simulink model "rst_auto_reg_complete_2018b"  (R2018b)
settings: Solver=VariableStepAuto  StartTime=0.0  StopTime=100  RelTol=1e-3
values from neighbouring files (symbols this model uses):
  A = dend    [RST_2ordem_final.m]    (also in RST_4ordem_final.m)
  B = numd    [RST_2ordem_final.m]    (also in RST_4ordem_final.m)
  ep = 0.7    [RST_2ordem_final.m]    (also in RST_4ordem_final.m)
  initial_theta = [-0.31 -0.55 0.0021 0.12]    [RST_2ordem_final.m]    (also in RST_4ordem_final.m = [-1.0 0.38 0.07 0.23 0.03 0.12 0.06 0.005])
  Ta = 0.1    [RST_2ordem_final.m]    (also in RST_4ordem_final.m = 1)
  Tas = Ta    (= 0.1)    [RST_2ordem_final.m]    (also in RST_4ordem_final.m = 1)
  theta_switch_time = 10*Ta    (= 1)    [RST_2ordem_final.m]    (also in RST_4ordem_final.m = 10)
  Ts = 1    [RST_2ordem_final.m]    (also in RST_4ordem_final.m = 5)
  w0 = 1    [RST_2ordem_final.m]    (also in RST_4ordem_final.m = 0.1)
libraries: dspinverses x6, simulink x1
settings Model: Creator=tarci  LastModifiedBy=root
settings DebuggingCC: LibraryContextMissingDiagnostic=none
settings SFSimCC: SimUseLocalCustomCode=off
settings RTWCC: RTWUseLocalCustomCode=off

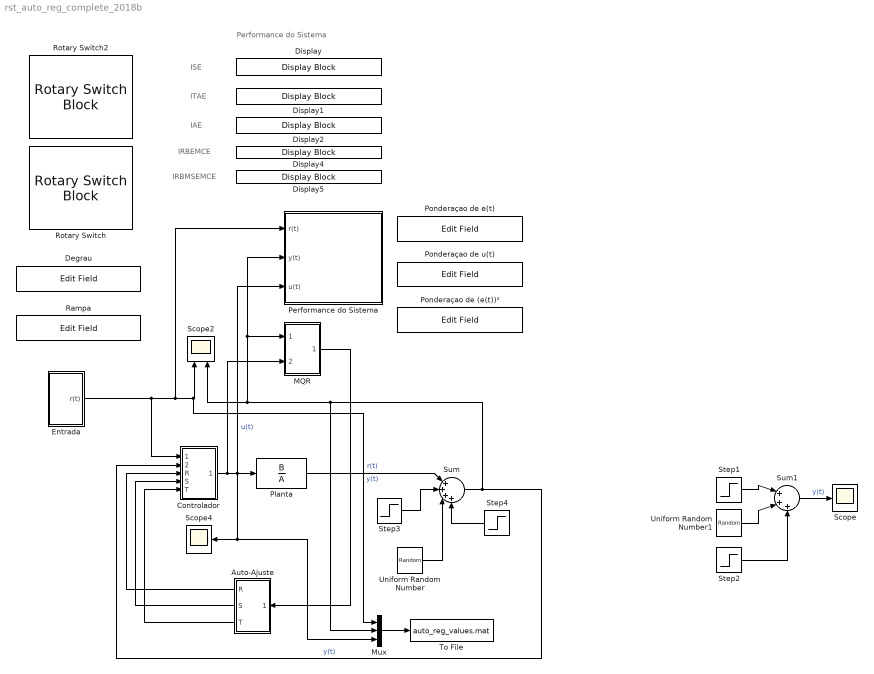
== system rst_auto_reg_complete_2018b ==
  note: ISE
  note: Performance do Sistema
  note: ITAE
  note: IAE
  note: IRBEMCE
  note: IRBMSEMCE
  Auto-Ajuste : Subsystem
  Controlador : Subsystem
  Degrau : EditField  WebBlockId=1122  LabelPosition=Hide  ShowInitialText=on  Alignment=Center
  Display : DisplayBlock  WebBlockId=1210  LabelPosition=Hide
  Display1 : DisplayBlock  WebBlockId=1211  LabelPosition=Hide
  Display2 : DisplayBlock  WebBlockId=1212  LabelPosition=Hide
  Display4 : DisplayBlock  WebBlockId=1214  LabelPosition=Hide
  Display5 : DisplayBlock  WebBlockId=1215  LabelPosition=Hide
  Entrada : Subsystem
  MQR : Subsystem
  Mux : Mux  Inputs=3
  Performance do Sistema : Subsystem
  Planta : DiscreteFilter  Numerator=B  Denominator=A  SampleTime=Ta  a0EqualsOne=on
  Ponderaçao de (e(t))² : EditField  WebBlockId=1158  LabelPosition=Hide  ShowInitialText=on  Alignment=Center
  Ponderaçao de e(t) : EditField  WebBlockId=1155  LabelPosition=Hide  ShowInitialText=on  Alignment=Center
  Ponderaçao de u(t) : EditField  WebBlockId=1156  LabelPosition=Hide  ShowInitialText=on  Alignment=Center
  Rampa : EditField  WebBlockId=1123  LabelPosition=Hide  ShowInitialText=on  Alignment=Center
  Rotary Switch : RotarySwitchBlock  WebBlockId=1169
      settings: Values={{'Degrau', 'Rampa', 'Senoide'}, [1 2 3]}
  Rotary Switch2 : RotarySwitchBlock  WebBlockId=1120
      settings: Values={{'Degrau', 'Rampa', 'Senoide'}, [1 2 3]}
  Scope : Scope
  Scope2 : Scope  NumInputPorts=2
  Scope4 : Scope
  Step1 : Step  Time=60  SampleTime=0
  Step2 : Step  Time=61  After=-1  SampleTime=0
  Step3 : Step  Time=60  SampleTime=0
  Step4 : Step  Time=61  After=-1  SampleTime=0
  Sum : Sum  Inputs=|++++
  Sum1 : Sum  Inputs=|+++
  To File : ToFile  Filename=auto_reg_values.mat
  Uniform Random Number : UniformRandomNumber  Minimum=-0.10  Maximum=0.10  Seed=10  SampleTime=0
  Uniform Random Number1 : UniformRandomNumber  Minimum=-0.10  Maximum=0.10  Seed=10  SampleTime=0
  wires:
  Auto-Ajuste/3(T) -> Controlador/5(T)
  Auto-Ajuste/1(R) -> Controlador/3(R)
  MQR/1("Theta(t) ") -> Auto-Ajuste/1(Theta)
  Entrada/1(r(t)) -> Mux/1, Scope2/1, Performance do Sistema/1(r(t)), Controlador/1(r(t))  "r(t)"
  Controlador/1(u(t)) -> Mux/3, Scope4/1, Performance do Sistema/3(u(t)), Planta/1, MQR/2("u(t) ")  "u(t)"
  Auto-Ajuste/2(S) -> Controlador/4(S)
  Mux/1 -> To File/1
  Step3/1 -> Sum/2
  Uniform Random Number/1 -> Sum/3
  Step4/1 -> Sum/4
  Planta/1 -> Sum/1  "y(t)"
  Sum/1 -> Mux/2, Scope2/2, Performance do Sistema/2(y(t)), MQR/1(y(t)), Controlador/2(y(t))  "y(t)"
  Uniform Random Number1/1 -> Sum1/2
  Step2/1 -> Sum1/3
  Step1/1 -> Sum1/1
  Sum1/1 -> Scope/1  "y(t)"

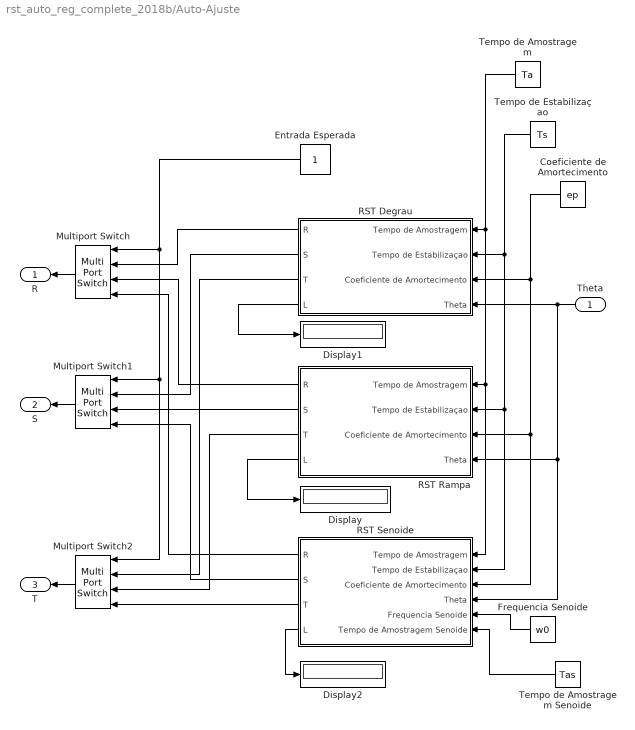
== system rst_auto_reg_complete_2018b/Auto-Ajuste ==
  Theta : Inport
  Coeficiente de Amortecimento : Constant  Value=ep
  Display : Display
  Display1 : Display
  Display2 : Display
  Entrada Esperada : Constant
  Frequencia Senoide : Constant  Value=w0
  Multiport Switch : MultiPortSwitch
  Multiport Switch1 : MultiPortSwitch
  Multiport Switch2 : MultiPortSwitch
  RST Degrau : Subsystem
  RST Rampa : Subsystem
  RST Senoide : Subsystem
  Tempo de Amostragem : Constant  Value=Ta
  Tempo de Amostragem Senoide : Constant  Value=Tas
  Tempo de Estabilizaçao : Constant  Value=Ts
  R : Outport
  S : Outport  Port=2
  T : Outport  Port=3
  wires:
  Entrada Esperada/1 -> Multiport Switch1/1, Multiport Switch2/1, Multiport Switch/1
  RST Degrau/1(R) -> Multiport Switch/2
  Coeficiente de Amortecimento/1 -> RST Senoide/3(Coeficiente de Amortecimento), RST Rampa/3(Coeficiente de Amortecimento), RST Degrau/3(Coeficiente de Amortecimento)
  RST Degrau/3(T) -> Multiport Switch2/2
  Theta/1 -> RST Senoide/4(Theta), RST Rampa/4(Theta), RST Degrau/4(Theta)
  RST Rampa/3(T) -> Multiport Switch2/3
  Tempo de Amostragem/1 -> RST Senoide/1(Tempo de Amostragem), RST Rampa/1(Tempo de Amostragem), RST Degrau/1(Tempo de Amostragem)
  Tempo de Amostragem Senoide/1 -> RST Senoide/6(Tempo de Amostragem Senoide)
  Frequencia Senoide/1 -> RST Senoide/5(Frequencia Senoide)
  RST Rampa/1(R) -> Multiport Switch/3
  RST Senoide/2(S) -> Multiport Switch1/4
  RST Degrau/2(S) -> Multiport Switch1/2
  Tempo de Estabilizaçao/1 -> RST Senoide/2(Tempo de Estabilizaçao), RST Rampa/2(Tempo de Estabilizaçao), RST Degrau/2(Tempo de Estabilizaçao)
  RST Senoide/1(R) -> Multiport Switch/4
  Multiport Switch/1 -> R/1
  Multiport Switch1/1 -> S/1
  Multiport Switch2/1 -> T/1
  RST Rampa/4(L) -> Display/1
  RST Senoide/3(T) -> Multiport Switch2/4
  RST Rampa/2(S) -> Multiport Switch1/3
  RST Degrau/4(L) -> Display1/1
  RST Senoide/4(L) -> Display2/1

== system rst_auto_reg_complete_2018b/Controlador ==
  r(t) : Inport
  y(t) : Inport  Port=2
  R : Inport  Port=3
  S : Inport  Port=4
  T : Inport  Port=5
  1/S3 : DiscreteFilter  Numerator=1  DenominatorSource=Input port  Denominator=1  SampleTime=Ta  a0EqualsOne=on
      settings: InputPortMap=u0,p3
  R3 : DiscreteFilter  NumeratorSource=Input port  Numerator=[-620.2 131.3]  Denominator=1  SampleTime=Ta
      settings: InputPortMap=u0,p1
  Sum11 : Sum  Inputs=|+-
  T3 : DiscreteFilter  NumeratorSource=Input port  Numerator=13.39  Denominator=1  SampleTime=Ta
      settings: InputPortMap=u0,p1
  u(t) : Outport
  wires:
  T3/1 -> Sum11/1
  T/1 -> T3/2
  Sum11/1 -> 1/S3/1
  R3/1 -> Sum11/2
  R/1 -> R3/2
  S/1 -> 1/S3/2
  r(t)/1 -> T3/1
  y(t)/1 -> R3/1
  1/S3/1 -> u(t)/1  "u(t)"

== system rst_auto_reg_complete_2018b/Entrada ==
  Multiport Switch : MultiPortSwitch
  Ramp : simulink/Sources/Ramp  slope=1  start=0  InitialOutput=0
  Sine Wave : Sin  Frequency=w0  SampleTime=Tas
  Step1 : Step  Time=0  SampleTime=0
  Step2 : Step  Time=10  After=2  SampleTime=0
  Step3 : Step  Time=20  After=-3  SampleTime=0
  Step4 : Step  Time=30  After=4  SampleTime=0
  Step5 : Step  Time=50  After=-2  SampleTime=0
  Sum : Sum  Inputs=|+++++
  Tipo de Entrada : Constant
  r(t) : Outport
  wires:
  Sine Wave/1 -> Multiport Switch/4
  Ramp/1 -> Multiport Switch/3
  Tipo de Entrada/1 -> Multiport Switch/1
  Multiport Switch/1 -> r(t)/1
  Step1/1 -> Sum/1
  Step2/1 -> Sum/2
  Step3/1 -> Sum/3
  Step4/1 -> Sum/4
  Sum/1 -> Multiport Switch/2
  Step5/1 -> Sum/5

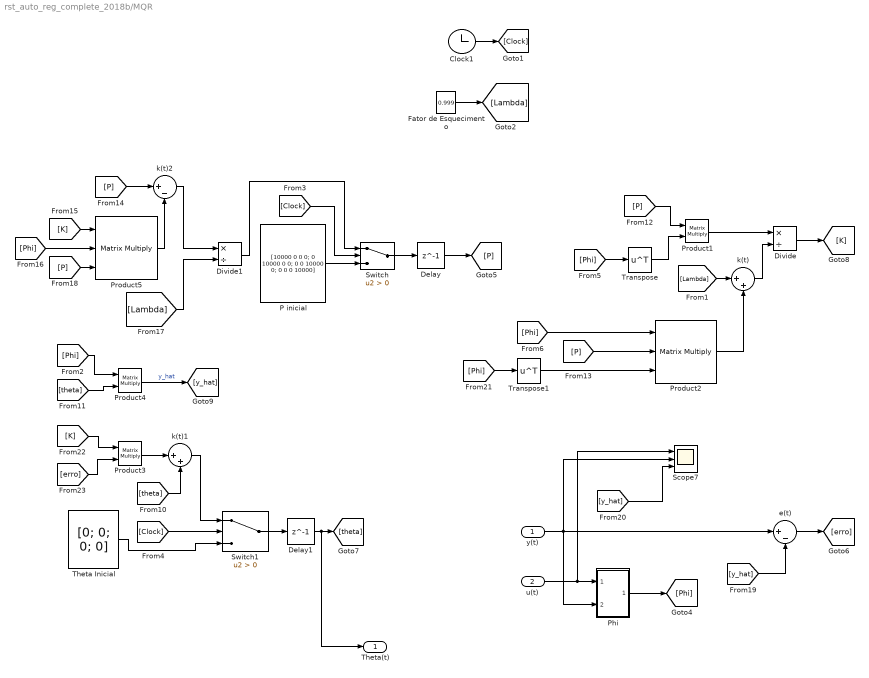
== system rst_auto_reg_complete_2018b/MQR ==
  y(t) : Inport
  "u(t) " : Inport  Port=2
  Clock1 : Clock
  Delay : Delay  DelayLength=1  InitialCondition=0
  Delay1 : Delay  DelayLength=1  InitialCondition=0
  Divide : Product  Inputs=*/
  Divide1 : Product  Inputs=*/
  "Fator de Esquecimento " : Constant  Value=0.999
  P inicial : Constant  Value=[10000 0 0 0; 0 10000 0 0; 0 0 10000 0; 0 0 0 10000]
  Phi : Subsystem
  Product1 : Product  Multiplication=Matrix(*)
  Product2 : Product  Inputs=3  Multiplication=Matrix(*)
  Product3 : Product  Multiplication=Matrix(*)
  Product4 : Product  Multiplication=Matrix(*)
  Product5 : Product  Inputs=3  Multiplication=Matrix(*)
  Scope7 : Scope  NumInputPorts=3
  Switch : Switch  Criteria=u2 > Threshold
  Switch1 : Switch  Criteria=u2 > Threshold
  "Theta Inicial " : Constant  Value=[0; 0; 0; 0]
  Transpose : Math  Operator=transpose  SaturateOnIntegerOverflow=on
  Transpose1 : Math  Operator=transpose  SaturateOnIntegerOverflow=on
  e(t) : Sum  Inputs=|+-
  k(t) : Sum  Inputs=|++
  k(t)1 : Sum  Inputs=|++
  k(t)2 : Sum  Inputs=|+-
  "Theta(t) " : Outport
  wires:
  k(t)/1 -> Divide/2
  [Phi] -> Product4/1
  Phi/1(Phi) -> [Phi]
  k(t)1/1 -> Switch1/1
  [y_hat] -> Scope7/3
  Switch1/1 -> Delay1/1
  [K] -> Product3/1
  Product2/1 -> k(t)/2
  [Clock] -> Switch1/2
  y(t)/1 -> e(t)/1, Scope7/2, Phi/2(y(t))
  k(t)2/1 -> Divide1/1
  Delay1/1 -> "Theta(t) "/1, [theta]
  Product5/1 -> k(t)2/2
  "u(t) "/1 -> Scope7/1, Phi/1(u(t))
  Switch/1 -> Delay/1
  [Lambda] -> Divide1/2
  Product1/1 -> Divide/1
  e(t)/1 -> [erro]
  Product3/1 -> k(t)1/1
  Delay/1 -> [P]
  [Phi] -> Transpose1/1
  [P] -> Product5/3
  "Fator de Esquecimento "/1 -> [Lambda]
  "Theta Inicial "/1 -> Switch1/3
  Transpose1/1 -> Product2/3
  Divide1/1 -> Switch/1
  [Phi] -> Transpose/1
  [Clock] -> Switch/2
  [theta] -> Product4/2
  [P] -> k(t)2/1
  [theta] -> k(t)1/2
  [P] -> Product2/2
  [Lambda] -> k(t)/1
  Transpose/1 -> Product1/2
  Clock1/1 -> [Clock]
  [erro] -> Product3/2
  [y_hat] -> e(t)/2
  [K] -> Product5/1
  P inicial/1 -> Switch/3
  [P] -> Product1/1
  [Phi] -> Product2/1
  Divide/1 -> [K]
  [Phi] -> Product5/2
  Product4/1 -> [y_hat]  "y_hat"

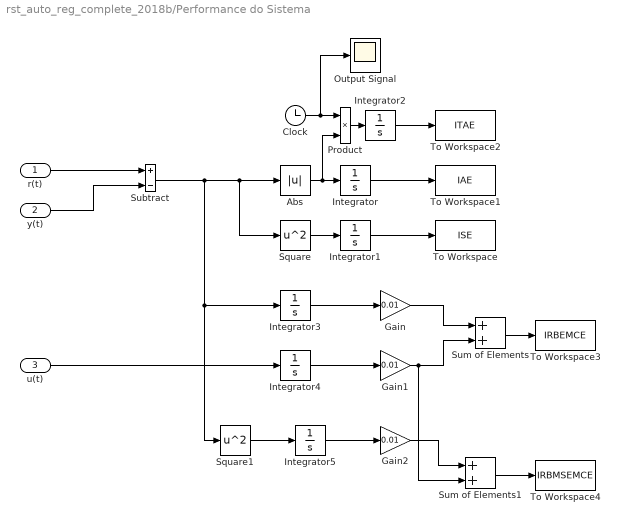
== system rst_auto_reg_complete_2018b/Performance do Sistema ==
  r(t) : Inport
  y(t) : Inport  Port=2
  u(t) : Inport  Port=3
  Abs : Abs
  Clock : Clock
  Gain : Gain  Gain=0.01
  Gain1 : Gain  Gain=0.01
  Gain2 : Gain  Gain=0.01
  Integrator{,1..5} (6 alike) : Integrator
  Output Signal : Scope
  Product : Product
  Square : Math  Operator=square  SaturateOnIntegerOverflow=on
  Square1 : Math  Operator=square  SaturateOnIntegerOverflow=on
  Subtract : Sum  Inputs=+-
  Sum of Elements : Sum
  Sum of Elements1 : Sum
  To Workspace : ToWorkspace  VariableName=ISE  SaveFormat=Timeseries  SampleTime=-1
  To Workspace1 : ToWorkspace  VariableName=IAE  SaveFormat=Timeseries  SampleTime=-1
  To Workspace2 : ToWorkspace  VariableName=ITAE  SaveFormat=Timeseries  SampleTime=-1
  To Workspace3 : ToWorkspace  VariableName=IRBEMCE  SaveFormat=Timeseries  SampleTime=-1
  To Workspace4 : ToWorkspace  VariableName=IRBMSEMCE  SaveFormat=Timeseries  SampleTime=-1
  wires:
  y(t)/1 -> Subtract/2
  Abs/1 -> Product/2, Integrator/1
  Integrator/1 -> To Workspace1/1
  Integrator1/1 -> To Workspace/1
  Square/1 -> Integrator1/1
  Clock/1 -> Output Signal/1, Product/1
  Product/1 -> Integrator2/1
  Integrator2/1 -> To Workspace2/1
  r(t)/1 -> Subtract/1
  Subtract/1 -> Square1/1, Integrator3/1, Square/1, Abs/1
  Integrator3/1 -> Gain/1
  Integrator4/1 -> Gain1/1
  Gain/1 -> Sum of Elements/1
  Gain1/1 -> Sum of Elements1/2, Sum of Elements/2
  Square1/1 -> Integrator5/1
  Integrator5/1 -> Gain2/1
  Gain2/1 -> Sum of Elements1/1
  Sum of Elements/1 -> To Workspace3/1
  Sum of Elements1/1 -> To Workspace4/1
  u(t)/1 -> Integrator4/1

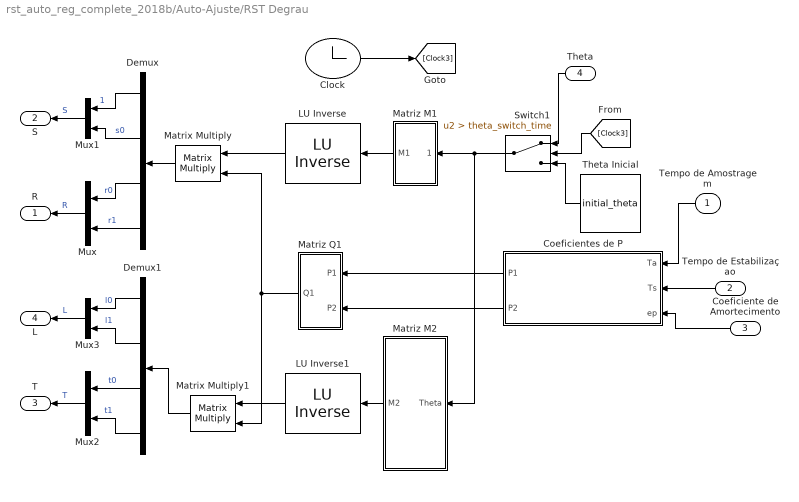
== system rst_auto_reg_complete_2018b/Auto-Ajuste/RST Degrau ==
  Tempo de Amostragem : Inport
  Tempo de Estabilizaçao : Inport  Port=2
  Coeficiente de Amortecimento : Inport  Port=3
  Theta : Inport  Port=4
  " LU Inverse" : dspinverses/ LU Inverse
      settings: SourceProductName=DSP System Toolbox
  " LU Inverse1" : dspinverses/ LU Inverse
      settings: SourceProductName=DSP System Toolbox
  Clock : Clock
  Coeficientes de P : Subsystem
  Demux : Demux
  Demux1 : Demux
  Matrix Multiply : Product  Multiplication=Matrix(*)
  Matrix Multiply1 : Product  Multiplication=Matrix(*)
  Matriz M1 : Subsystem
  Matriz M2 : Subsystem
  Matriz Q1 : Subsystem
  Mux{,1..3} (4 alike) : Mux  Inputs=2
  Switch1 : Switch  Criteria=u2 > Threshold  Threshold=theta_switch_time
  Theta Inicial : Constant  Value=initial_theta
  R : Outport
  S : Outport  Port=2
  T : Outport  Port=3
  L : Outport  Port=4
  wires:
  Matrix Multiply/1 -> Demux/1
  " LU Inverse"/1 -> Matrix Multiply/1
  Mux1/1 -> S/1  "S"
  Coeficientes de P/2(P2) -> Matriz Q1/2(P2)
  Tempo de Estabilizaçao/1 -> Coeficientes de P/2(Ts)
  Coeficiente de Amortecimento/1 -> Coeficientes de P/3(ep)
  Tempo de Amostragem/1 -> Coeficientes de P/1(Ta)
  Coeficientes de P/1(P1) -> Matriz Q1/1(P1)
  Mux/1 -> R/1  "R"
  Clock/1 -> [Clock3]
  Switch1/1 -> Matriz M2/1(Theta), Matriz M1/1(In1)
  Theta/1 -> Switch1/1
  [Clock3] -> Switch1/2
  Theta Inicial/1 -> Switch1/3
  Matriz M1/1(M1) -> " LU Inverse"/1
  Demux/1 -> Mux1/1  "1"
  Demux/2 -> Mux1/2  "s0"
  Demux/3 -> Mux/1  "r0"
  Demux/4 -> Mux/2  "r1"
  " LU Inverse1"/1 -> Matrix Multiply1/1
  Matriz Q1/1(Q1) -> Matrix Multiply/2, Matrix Multiply1/2
  Matriz M2/1(M2) -> " LU Inverse1"/1
  Demux1/3 -> Mux2/1  "t0"
  Mux2/1 -> T/1  "T"
  Demux1/2 -> Mux3/2  "l1"
  Mux3/1 -> L/1  "L"
  Demux1/1 -> Mux3/1  "l0"
  Matrix Multiply1/1 -> Demux1/1
  Demux1/4 -> Mux2/2  "t1"

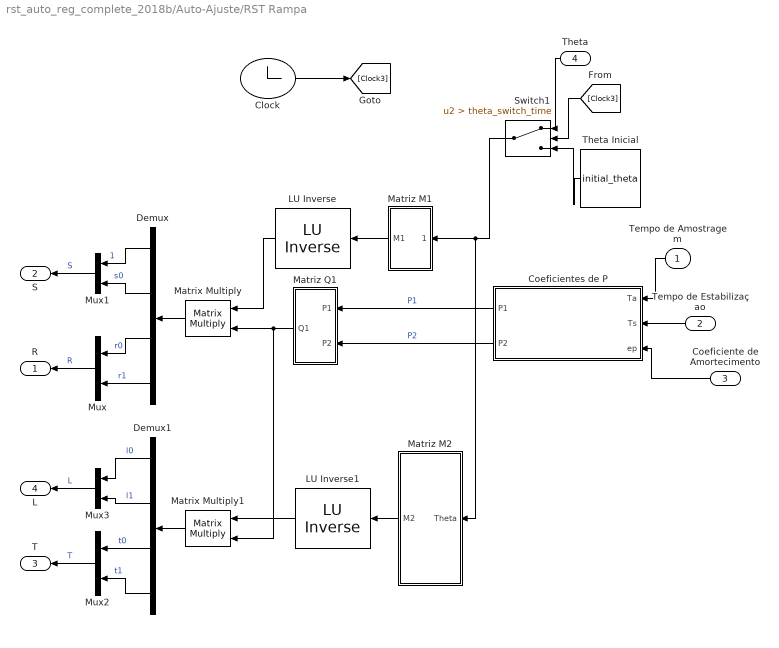
== system rst_auto_reg_complete_2018b/Auto-Ajuste/RST Rampa ==
  Tempo de Amostragem : Inport
  Tempo de Estabilizaçao : Inport  Port=2
  Coeficiente de Amortecimento : Inport  Port=3
  Theta : Inport  Port=4
  " LU Inverse" : dspinverses/ LU Inverse
      settings: SourceProductName=DSP System Toolbox
  " LU Inverse1" : dspinverses/ LU Inverse
      settings: SourceProductName=DSP System Toolbox
  Clock : Clock
  Coeficientes de P : Subsystem
  Demux : Demux
  Demux1 : Demux
  Matrix Multiply : Product  Multiplication=Matrix(*)
  Matrix Multiply1 : Product  Multiplication=Matrix(*)
  Matriz M1 : Subsystem
  Matriz M2 : Subsystem
  Matriz Q1 : Subsystem
  Mux{,1..3} (4 alike) : Mux  Inputs=2
  Switch1 : Switch  Criteria=u2 > Threshold  Threshold=theta_switch_time
  Theta Inicial : Constant  Value=initial_theta
  R : Outport
  S : Outport  Port=2
  T : Outport  Port=3
  L : Outport  Port=4
  wires:
  Demux/4 -> Mux/2  "r1"
  Demux/3 -> Mux/1  "r0"
  Demux/2 -> Mux1/2  "s0"
  Demux/1 -> Mux1/1  "1"
  Matriz Q1/1(Q1) -> Matrix Multiply/2, Matrix Multiply1/2
  Matriz M1/1(M1) -> " LU Inverse"/1
  Theta Inicial/1 -> Switch1/3
  [Clock3] -> Switch1/2
  Theta/1 -> Switch1/1
  Switch1/1 -> Matriz M2/1(Theta), Matriz M1/1(In1)
  Clock/1 -> [Clock3]
  Mux/1 -> R/1  "R"
  Coeficientes de P/1(P1) -> Matriz Q1/1(P1)  "P1"
  Tempo de Amostragem/1 -> Coeficientes de P/1(Ta)
  Coeficiente de Amortecimento/1 -> Coeficientes de P/3(ep)
  Tempo de Estabilizaçao/1 -> Coeficientes de P/2(Ts)
  Coeficientes de P/2(P2) -> Matriz Q1/2(P2)  "P2"
  Mux1/1 -> S/1  "S"
  " LU Inverse"/1 -> Matrix Multiply/1
  Matrix Multiply/1 -> Demux/1
  Matriz M2/1(M2) -> " LU Inverse1"/1
  " LU Inverse1"/1 -> Matrix Multiply1/1
  Mux3/1 -> L/1  "L"
  Mux2/1 -> T/1  "T"
  Demux1/1 -> Mux3/1  "l0"
  Demux1/2 -> Mux3/2  "l1"
  Demux1/3 -> Mux2/1  "t0"
  Demux1/4 -> Mux2/2  "t1"
  Matrix Multiply1/1 -> Demux1/1

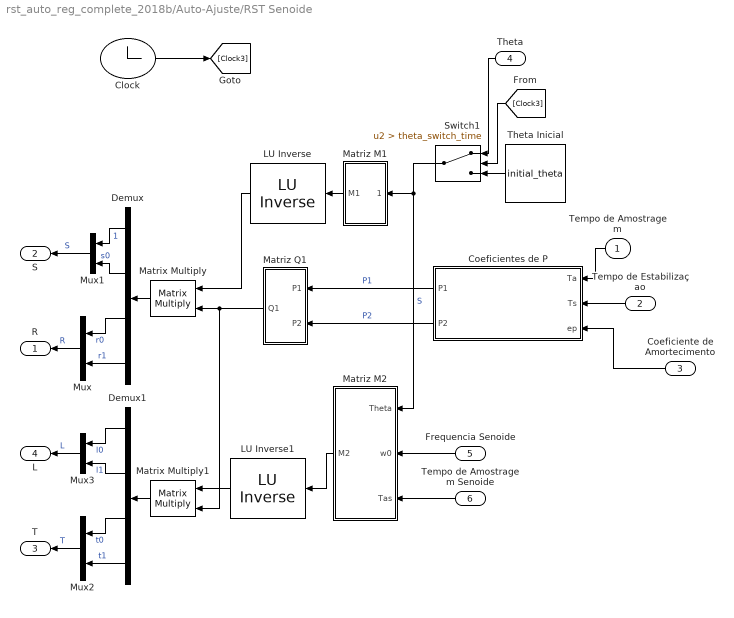
== system rst_auto_reg_complete_2018b/Auto-Ajuste/RST Senoide ==
  Tempo de Amostragem : Inport
  Tempo de Estabilizaçao : Inport  Port=2
  Coeficiente de Amortecimento : Inport  Port=3
  Theta : Inport  Port=4
  Frequencia Senoide : Inport  Port=5
  Tempo de Amostragem Senoide : Inport  Port=6
  " LU Inverse" : dspinverses/ LU Inverse
      settings: SourceProductName=DSP System Toolbox
  " LU Inverse1" : dspinverses/ LU Inverse
      settings: SourceProductName=DSP System Toolbox
  Clock : Clock
  Coeficientes de P : Subsystem
  Demux : Demux
  Demux1 : Demux
  Matrix Multiply : Product  Multiplication=Matrix(*)
  Matrix Multiply1 : Product  Multiplication=Matrix(*)
  Matriz M1 : Subsystem
  Matriz M2 : Subsystem
  Matriz Q1 : Subsystem
  Mux{,1..3} (4 alike) : Mux  Inputs=2
  Switch1 : Switch  Criteria=u2 > Threshold  Threshold=theta_switch_time
  Theta Inicial : Constant  Value=initial_theta
  R : Outport
  S : Outport  Port=2
  T : Outport  Port=3
  L : Outport  Port=4
  wires:
  Demux/4 -> Mux/2  "r1"
  Demux/3 -> Mux/1  "r0"
  Demux/2 -> Mux1/2  "s0"
  Demux/1 -> Mux1/1  "1"
  Matriz Q1/1(Q1) -> Matrix Multiply/2, Matrix Multiply1/2
  Matriz M1/1(M1) -> " LU Inverse"/1
  Theta Inicial/1 -> Switch1/3
  [Clock3] -> Switch1/2
  Theta/1 -> Switch1/1
  Switch1/1 -> Matriz M2/1(Theta), Matriz M1/1(In1)  "S"
  Clock/1 -> [Clock3]
  Mux/1 -> R/1  "R"
  Coeficientes de P/1(P1) -> Matriz Q1/1(P1)  "P1"
  Tempo de Amostragem/1 -> Coeficientes de P/1(Ta)
  Coeficiente de Amortecimento/1 -> Coeficientes de P/3(ep)
  Tempo de Estabilizaçao/1 -> Coeficientes de P/2(Ts)
  Coeficientes de P/2(P2) -> Matriz Q1/2(P2)  "P2"
  Mux1/1 -> S/1  "S"
  " LU Inverse"/1 -> Matrix Multiply/1
  Matrix Multiply/1 -> Demux/1
  Frequencia Senoide/1 -> Matriz M2/2(w0)
  Tempo de Amostragem Senoide/1 -> Matriz M2/3(Tas)
  Matriz M2/1(M2) -> " LU Inverse1"/1
  " LU Inverse1"/1 -> Matrix Multiply1/1
  Mux3/1 -> L/1  "L"
  Mux2/1 -> T/1  "T"
  Demux1/1 -> Mux3/1  "l0"
  Demux1/2 -> Mux3/2  "l1"
  Demux1/3 -> Mux2/1  "t0"
  Demux1/4 -> Mux2/2  "t1"
  Matrix Multiply1/1 -> Demux1/1

== system rst_auto_reg_complete_2018b/MQR/Phi ==
  u(t) : Inport
  y(t) : Inport  Port=2
  Constant : Constant  Value=-1
  Delay : Delay
  Delay1 : Delay  DelayLength=1
  Delay2 : Delay
  Delay3 : Delay  DelayLength=1
  Product : Product
  Transpose1 : Math  Operator=transpose  SaturateOnIntegerOverflow=on
  Vector Concatenate : Concatenate  NumInputs=4
  Phi : Outport
  wires:
  u(t)/1 -> Delay2/1, Delay3/1
  Vector Concatenate/1 -> Transpose1/1  "Phi"
  Delay/1 -> Vector Concatenate/2
  y(t)/1 -> Product/1
  Delay3/1 -> Vector Concatenate/3
  Delay2/1 -> Vector Concatenate/4
  Delay1/1 -> Vector Concatenate/1
  Transpose1/1 -> Phi/1
  Constant/1 -> Product/2
  Product/1 -> Delay/1, Delay1/1

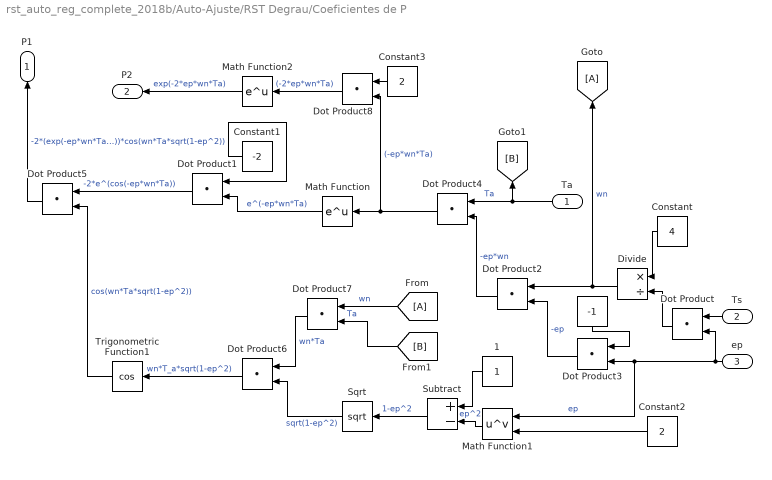
== system rst_auto_reg_complete_2018b/Auto-Ajuste/RST Degrau/Coeficientes de P ==
  Ta : Inport
  Ts : Inport  Port=2
  ep : Inport  Port=3
  " " : Constant  Value=-1
  1 : Constant
  Constant : Constant  Value=4
  Constant1 : Constant  Value=-2
  Constant2 : Constant  Value=2
  Constant3 : Constant  Value=2
  Divide : Product  Inputs=*/
  Dot Product{,1..8} (9 alike) : DotProduct  InputSameDT=on  OutDataTypeStr=Inherit: Inherit via internal rule
  Math Function : Math  SaturateOnIntegerOverflow=on
  Math Function1 : Math  Operator=pow  SaturateOnIntegerOverflow=on
  Math Function2 : Math  SaturateOnIntegerOverflow=on
  Sqrt : Sqrt  SaturateOnIntegerOverflow=on
  Subtract : Sum  Inputs=+-
  Trigonometric Function1 : Trigonometry  Operator=cos
  P1 : Outport
  P2 : Outport  Port=2
  wires:
  Math Function/1 -> Dot Product1/2  "e^(-ep*wn*Ta)"
  Divide/1 -> Dot Product2/1, [A]  "wn"
  [A] -> Dot Product7/1  "wn"
  " "/1 -> Dot Product3/1
  Dot Product5/1 -> P1/1  "-2*(exp(-ep*wn*Ta))*cos(wn*Ta*sqrt(1-ep^2))"
  Trigonometric Function1/1 -> Dot Product5/2  "cos(wn*Ta*sqrt(1-ep^2))"
  Ts/1 -> Dot Product/1
  Dot Product/1 -> Divide/2
  Dot Product3/1 -> Dot Product2/2  "-ep"
  ep/1 -> Math Function1/1, Dot Product3/2, Dot Product/2  "ep"
  Constant/1 -> Divide/1
  Dot Product7/1 -> Dot Product6/1  "wn*Ta"
  Ta/1 -> Dot Product4/1, [B]  "Ta"
  Math Function1/1 -> Subtract/2  "ep^2"
  Dot Product1/1 -> Dot Product5/1  "-2*e^(cos(-ep*wn*Ta))"
  Constant2/1 -> Math Function1/2
  1/1 -> Subtract/1
  Constant1/1 -> Dot Product1/1
  Dot Product2/1 -> Dot Product4/2  "-ep*wn"
  [B] -> Dot Product7/2  "Ta"
  Dot Product6/1 -> Trigonometric Function1/1  "wn*T_a*sqrt(1-ep^2)"
  Dot Product4/1 -> Dot Product8/2, Math Function/1  "(-ep*wn*Ta)"
  Sqrt/1 -> Dot Product6/2  "sqrt(1-ep^2)"
  Subtract/1 -> Sqrt/1  "1-ep^2"
  Constant3/1 -> Dot Product8/1
  Dot Product8/1 -> Math Function2/1  "(-2*ep*wn*Ta)"
  Math Function2/1 -> P2/1  "exp(-2*ep*wn*Ta)"

== system rst_auto_reg_complete_2018b/Auto-Ajuste/RST Degrau/Matriz M1 ==
  In1 : Inport
  " 1" : Constant  Value=0
  2 : Constant
  Demux : Demux
  Matrix Concatenate{6,9..11} (4 alike) : Concatenate  NumInputs=4  Mode=Multidimensional array  ConcatenateDimension=2
  Matrix Concatenate12 : Concatenate  Mode=Multidimensional array
  Matrix Concatenate13 : Concatenate  Mode=Multidimensional array
  Matrix Concatenate14 : Concatenate  Mode=Multidimensional array
  M1 : Outport
  wires:
  In1/1 -> Demux/1
  Demux/3 -> Matrix Concatenate9/3, Matrix Concatenate10/4  "b1"
  Matrix Concatenate14/1 -> M1/1
  Demux/1 -> Matrix Concatenate10/2, Matrix Concatenate9/1  "a1"
  Demux/4 -> Matrix Concatenate10/3, Matrix Concatenate11/4  "b2"
  Demux/2 -> Matrix Concatenate11/2, Matrix Concatenate10/1  "a2"
  2/1 -> Matrix Concatenate9/2, Matrix Concatenate6/1  "1"
  " 1"/1 -> Matrix Concatenate6/3, Matrix Concatenate11/3, Matrix Concatenate11/1, Matrix Concatenate9/4, Matrix Concatenate6/4, Matrix Concatenate6/2  "0"
  Matrix Concatenate6/1 -> Matrix Concatenate12/1
  Matrix Concatenate9/1 -> Matrix Concatenate12/2
  Matrix Concatenate10/1 -> Matrix Concatenate13/1
  Matrix Concatenate11/1 -> Matrix Concatenate13/2
  Matrix Concatenate13/1 -> Matrix Concatenate14/2
  Matrix Concatenate12/1 -> Matrix Concatenate14/1

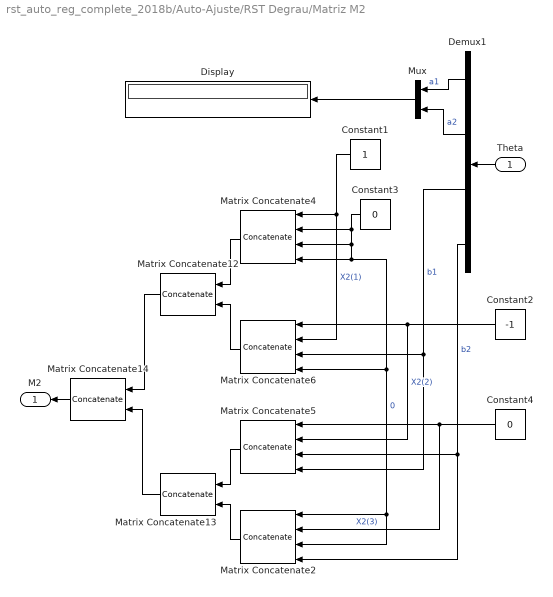
== system rst_auto_reg_complete_2018b/Auto-Ajuste/RST Degrau/Matriz M2 ==
  Theta : Inport
  Constant1 : Constant
  Constant2 : Constant  Value=-1
  Constant3 : Constant  Value=0
  Constant4 : Constant  Value=0
  Demux1 : Demux
  Display : Display
  Matrix Concatenate12 : Concatenate  Mode=Multidimensional array
  Matrix Concatenate13 : Concatenate  Mode=Multidimensional array
  Matrix Concatenate14 : Concatenate  Mode=Multidimensional array
  Matrix Concatenate{2,4..6} (4 alike) : Concatenate  NumInputs=4  Mode=Multidimensional array  ConcatenateDimension=2
  Mux : Mux  Inputs=2
  M2 : Outport
  wires:
  Matrix Concatenate6/1 -> Matrix Concatenate12/2
  Theta/1 -> Demux1/1
  Constant1/1 -> Matrix Concatenate6/2, Matrix Concatenate4/1  "X2(1)"
  Constant3/1 -> Matrix Concatenate4/3, Matrix Concatenate2/3, Matrix Concatenate2/1, Matrix Concatenate6/4, Matrix Concatenate4/4, Matrix Concatenate4/2  "0"
  Demux1/3 -> Matrix Concatenate5/4, Matrix Concatenate6/3  "b1"
  Demux1/4 -> Matrix Concatenate2/4, Matrix Concatenate5/3  "b2"
  Matrix Concatenate14/1 -> M2/1
  Matrix Concatenate13/1 -> Matrix Concatenate14/2
  Matrix Concatenate12/1 -> Matrix Concatenate14/1
  Matrix Concatenate4/1 -> Matrix Concatenate12/1
  Matrix Concatenate5/1 -> Matrix Concatenate13/1
  Matrix Concatenate2/1 -> Matrix Concatenate13/2
  Constant2/1 -> Matrix Concatenate5/2, Matrix Concatenate6/1  "X2(2)"
  Constant4/1 -> Matrix Concatenate2/2, Matrix Concatenate5/1  "X2(3)"
  Mux/1 -> Display/1
  Demux1/1 -> Mux/1  "a1"
  Demux1/2 -> Mux/2  "a2"

== system rst_auto_reg_complete_2018b/Auto-Ajuste/RST Degrau/Matriz Q1 ==
  P1 : Inport
  P2 : Inport  Port=2
  Constant : Constant
  Constant1 : Constant  Value=0
  Matrix Concatenate1 : Concatenate  Mode=Multidimensional array
  Matrix Concatenate2 : Concatenate  Mode=Multidimensional array
  Matrix Concatenate3 : Concatenate  Mode=Multidimensional array
  Q1 : Outport
  wires:
  Matrix Concatenate1/1 -> Matrix Concatenate2/1
  Matrix Concatenate2/1 -> Q1/1
  Matrix Concatenate3/1 -> Matrix Concatenate2/2
  P2/1 -> Matrix Concatenate3/1
  P1/1 -> Matrix Concatenate1/2
  Constant/1 -> Matrix Concatenate1/1
  Constant1/1 -> Matrix Concatenate3/2

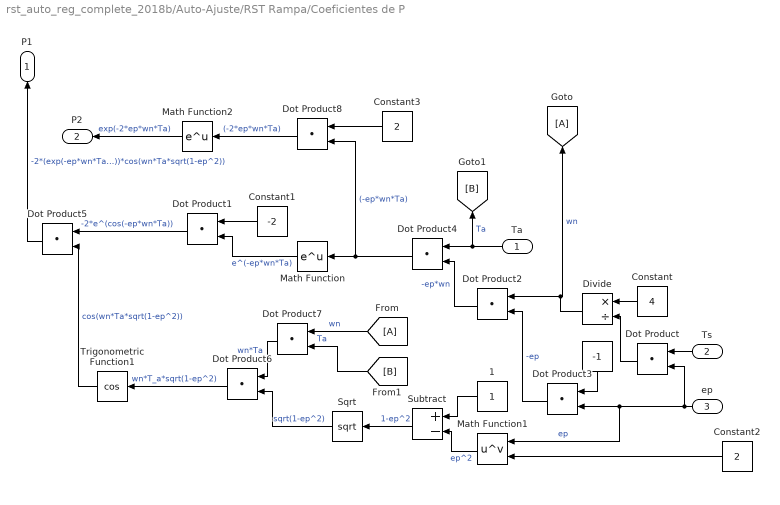
== system rst_auto_reg_complete_2018b/Auto-Ajuste/RST Rampa/Coeficientes de P ==
  Ta : Inport
  Ts : Inport  Port=2
  ep : Inport  Port=3
  " " : Constant  Value=-1
  1 : Constant
  Constant : Constant  Value=4
  Constant1 : Constant  Value=-2
  Constant2 : Constant  Value=2
  Constant3 : Constant  Value=2
  Divide : Product  Inputs=*/
  Dot Product{,1..8} (9 alike) : DotProduct  InputSameDT=on  OutDataTypeStr=Inherit: Inherit via internal rule
  Math Function : Math  SaturateOnIntegerOverflow=on
  Math Function1 : Math  Operator=pow  SaturateOnIntegerOverflow=on
  Math Function2 : Math  SaturateOnIntegerOverflow=on
  Sqrt : Sqrt  SaturateOnIntegerOverflow=on
  Subtract : Sum  Inputs=+-
  Trigonometric Function1 : Trigonometry  Operator=cos
  P1 : Outport
  P2 : Outport  Port=2
  wires:
  Math Function2/1 -> P2/1  "exp(-2*ep*wn*Ta)"
  Dot Product8/1 -> Math Function2/1  "(-2*ep*wn*Ta)"
  Constant3/1 -> Dot Product8/1
  Subtract/1 -> Sqrt/1  "1-ep^2"
  Sqrt/1 -> Dot Product6/2  "sqrt(1-ep^2)"
  Dot Product4/1 -> Math Function/1, Dot Product8/2  "(-ep*wn*Ta)"
  Dot Product6/1 -> Trigonometric Function1/1  "wn*T_a*sqrt(1-ep^2)"
  [B] -> Dot Product7/2  "Ta"
  Dot Product2/1 -> Dot Product4/2  "-ep*wn"
  Constant1/1 -> Dot Product1/1
  1/1 -> Subtract/1
  Constant2/1 -> Math Function1/2
  Dot Product1/1 -> Dot Product5/1  "-2*e^(cos(-ep*wn*Ta))"
  Math Function1/1 -> Subtract/2  "ep^2"
  Ta/1 -> Dot Product4/1, [B]  "Ta"
  Dot Product7/1 -> Dot Product6/1  "wn*Ta"
  Constant/1 -> Divide/1
  ep/1 -> Dot Product/2, Dot Product3/2, Math Function1/1  "ep"
  Dot Product3/1 -> Dot Product2/2  "-ep"
  Dot Product/1 -> Divide/2
  Ts/1 -> Dot Product/1
  Trigonometric Function1/1 -> Dot Product5/2  "cos(wn*Ta*sqrt(1-ep^2))"
  Dot Product5/1 -> P1/1  "-2*(exp(-ep*wn*Ta))*cos(wn*Ta*sqrt(1-ep^2))"
  " "/1 -> Dot Product3/1
  [A] -> Dot Product7/1  "wn"
  Divide/1 -> [A], Dot Product2/1  "wn"
  Math Function/1 -> Dot Product1/2  "e^(-ep*wn*Ta)"

== system rst_auto_reg_complete_2018b/Auto-Ajuste/RST Rampa/Matriz M1 ==
  In1 : Inport
  " 1" : Constant  Value=0
  2 : Constant
  Demux : Demux
  Matrix Concatenate{6,9..11} (4 alike) : Concatenate  NumInputs=4  Mode=Multidimensional array  ConcatenateDimension=2
  Matrix Concatenate12 : Concatenate  Mode=Multidimensional array
  Matrix Concatenate13 : Concatenate  Mode=Multidimensional array
  Matrix Concatenate14 : Concatenate  Mode=Multidimensional array
  M1 : Outport
  wires:
  Matrix Concatenate12/1 -> Matrix Concatenate14/1
  Matrix Concatenate13/1 -> Matrix Concatenate14/2
  Matrix Concatenate11/1 -> Matrix Concatenate13/2
  Matrix Concatenate10/1 -> Matrix Concatenate13/1
  Matrix Concatenate9/1 -> Matrix Concatenate12/2
  Matrix Concatenate6/1 -> Matrix Concatenate12/1
  " 1"/1 -> Matrix Concatenate6/2, Matrix Concatenate6/4, Matrix Concatenate9/4, Matrix Concatenate11/1, Matrix Concatenate11/3, Matrix Concatenate6/3  "0"
  2/1 -> Matrix Concatenate6/1, Matrix Concatenate9/2  "1"
  Demux/2 -> Matrix Concatenate10/1, Matrix Concatenate11/2  "a2"
  Demux/4 -> Matrix Concatenate10/3, Matrix Concatenate11/4  "b2"
  Demux/1 -> Matrix Concatenate9/1, Matrix Concatenate10/2  "a1"
  Matrix Concatenate14/1 -> M1/1
  Demux/3 -> Matrix Concatenate9/3, Matrix Concatenate10/4  "b1"
  In1/1 -> Demux/1

== system rst_auto_reg_complete_2018b/Auto-Ajuste/RST Rampa/Matriz M2 ==
  Theta : Inport
  Constant1 : Constant
  Constant2 : Constant  Value=-2
  Constant3 : Constant  Value=0
  Constant4 : Constant
  Demux1 : Demux
  Display1 : Display
  Matrix Concatenate12 : Concatenate  Mode=Multidimensional array
  Matrix Concatenate13 : Concatenate  Mode=Multidimensional array
  Matrix Concatenate14 : Concatenate  Mode=Multidimensional array
  Matrix Concatenate{2,4..6} (4 alike) : Concatenate  NumInputs=4  Mode=Multidimensional array  ConcatenateDimension=2
  Mux : Mux  Inputs=2
  M2 : Outport
  wires:
  Matrix Concatenate6/1 -> Matrix Concatenate12/2
  Demux1/2 -> Mux/2  "a2"
  Theta/1 -> Demux1/1
  Demux1/1 -> Mux/1  "a1"
  Constant1/1 -> Matrix Concatenate6/2, Matrix Concatenate4/1  "X2(1)"
  Constant3/1 -> Matrix Concatenate4/3, Matrix Concatenate2/3, Matrix Concatenate2/1, Matrix Concatenate6/4, Matrix Concatenate4/4, Matrix Concatenate4/2  "0"
  Demux1/3 -> Matrix Concatenate5/4, Matrix Concatenate6/3  "b1"
  Demux1/4 -> Matrix Concatenate2/4, Matrix Concatenate5/3  "b2"
  Matrix Concatenate14/1 -> M2/1
  Matrix Concatenate13/1 -> Matrix Concatenate14/2
  Matrix Concatenate12/1 -> Matrix Concatenate14/1
  Matrix Concatenate4/1 -> Matrix Concatenate12/1
  Matrix Concatenate5/1 -> Matrix Concatenate13/1
  Matrix Concatenate2/1 -> Matrix Concatenate13/2
  Constant2/1 -> Matrix Concatenate5/2, Matrix Concatenate6/1  "X2(2)"
  Constant4/1 -> Matrix Concatenate2/2, Matrix Concatenate5/1  "X2(3)"
  Mux/1 -> Display1/1

== system rst_auto_reg_complete_2018b/Auto-Ajuste/RST Rampa/Matriz Q1 ==
  P1 : Inport
  P2 : Inport  Port=2
  Constant : Constant
  Constant1 : Constant  Value=0
  Matrix Concatenate1 : Concatenate  Mode=Multidimensional array
  Matrix Concatenate2 : Concatenate  Mode=Multidimensional array
  Matrix Concatenate3 : Concatenate  Mode=Multidimensional array
  Q1 : Outport
  wires:
  Constant1/1 -> Matrix Concatenate3/2
  Constant/1 -> Matrix Concatenate1/1
  P1/1 -> Matrix Concatenate1/2
  P2/1 -> Matrix Concatenate3/1
  Matrix Concatenate3/1 -> Matrix Concatenate2/2
  Matrix Concatenate2/1 -> Q1/1
  Matrix Concatenate1/1 -> Matrix Concatenate2/1

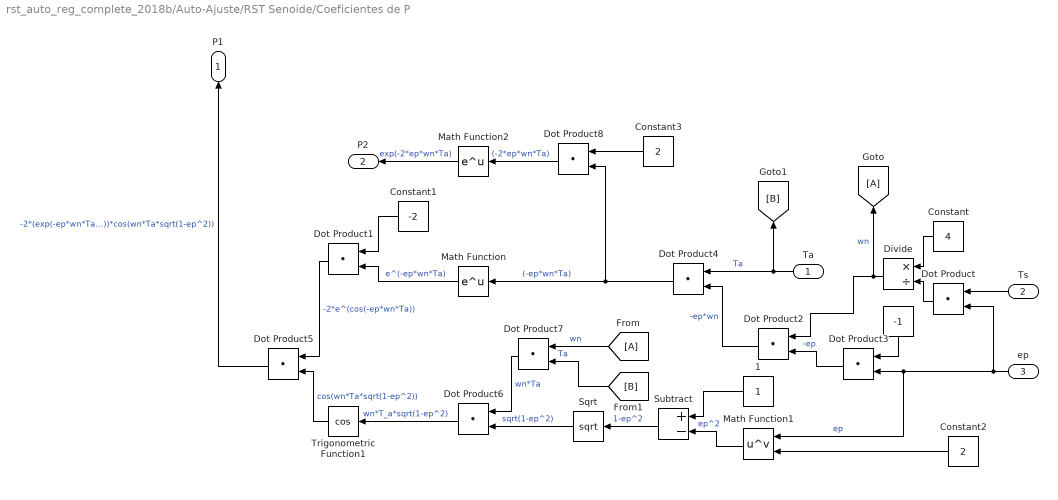
== system rst_auto_reg_complete_2018b/Auto-Ajuste/RST Senoide/Coeficientes de P ==
  Ta : Inport
  Ts : Inport  Port=2
  ep : Inport  Port=3
  " " : Constant  Value=-1
  1 : Constant
  Constant : Constant  Value=4
  Constant1 : Constant  Value=-2
  Constant2 : Constant  Value=2
  Constant3 : Constant  Value=2
  Divide : Product  Inputs=*/
  Dot Product{,1..8} (9 alike) : DotProduct  InputSameDT=on  OutDataTypeStr=Inherit: Inherit via internal rule
  Math Function : Math  SaturateOnIntegerOverflow=on
  Math Function1 : Math  Operator=pow  SaturateOnIntegerOverflow=on
  Math Function2 : Math  SaturateOnIntegerOverflow=on
  Sqrt : Sqrt  SaturateOnIntegerOverflow=on
  Subtract : Sum  Inputs=+-
  Trigonometric Function1 : Trigonometry  Operator=cos
  P1 : Outport
  P2 : Outport  Port=2
  wires:
  Math Function2/1 -> P2/1  "exp(-2*ep*wn*Ta)"
  Dot Product8/1 -> Math Function2/1  "(-2*ep*wn*Ta)"
  Constant3/1 -> Dot Product8/1
  Subtract/1 -> Sqrt/1  "1-ep^2"
  Sqrt/1 -> Dot Product6/2  "sqrt(1-ep^2)"
  Dot Product4/1 -> Math Function/1, Dot Product8/2  "(-ep*wn*Ta)"
  Dot Product6/1 -> Trigonometric Function1/1  "wn*T_a*sqrt(1-ep^2)"
  [B] -> Dot Product7/2  "Ta"
  Dot Product2/1 -> Dot Product4/2  "-ep*wn"
  Constant1/1 -> Dot Product1/1
  1/1 -> Subtract/1
  Constant2/1 -> Math Function1/2
  Dot Product1/1 -> Dot Product5/1  "-2*e^(cos(-ep*wn*Ta))"
  Math Function1/1 -> Subtract/2  "ep^2"
  Ta/1 -> Dot Product4/1, [B]  "Ta"
  Dot Product7/1 -> Dot Product6/1  "wn*Ta"
  Constant/1 -> Divide/1
  ep/1 -> Dot Product/2, Dot Product3/2, Math Function1/1  "ep"
  Dot Product3/1 -> Dot Product2/2  "-ep"
  Dot Product/1 -> Divide/2
  Ts/1 -> Dot Product/1
  Trigonometric Function1/1 -> Dot Product5/2  "cos(wn*Ta*sqrt(1-ep^2))"
  Dot Product5/1 -> P1/1  "-2*(exp(-ep*wn*Ta))*cos(wn*Ta*sqrt(1-ep^2))"
  " "/1 -> Dot Product3/1
  [A] -> Dot Product7/1  "wn"
  Divide/1 -> Dot Product2/1, [A]  "wn"
  Math Function/1 -> Dot Product1/2  "e^(-ep*wn*Ta)"

== system rst_auto_reg_complete_2018b/Auto-Ajuste/RST Senoide/Matriz M1 ==
  In1 : Inport
  " 1" : Constant  Value=0
  2 : Constant
  Demux : Demux
  Matrix Concatenate{6,9..11} (4 alike) : Concatenate  NumInputs=4  Mode=Multidimensional array  ConcatenateDimension=2
  Matrix Concatenate12 : Concatenate  Mode=Multidimensional array
  Matrix Concatenate13 : Concatenate  Mode=Multidimensional array
  Matrix Concatenate14 : Concatenate  Mode=Multidimensional array
  M1 : Outport
  wires:
  Matrix Concatenate12/1 -> Matrix Concatenate14/1
  Matrix Concatenate13/1 -> Matrix Concatenate14/2
  Matrix Concatenate11/1 -> Matrix Concatenate13/2
  Matrix Concatenate10/1 -> Matrix Concatenate13/1
  Matrix Concatenate9/1 -> Matrix Concatenate12/2
  Matrix Concatenate6/1 -> Matrix Concatenate12/1
  " 1"/1 -> Matrix Concatenate6/2, Matrix Concatenate6/4, Matrix Concatenate9/4, Matrix Concatenate11/1, Matrix Concatenate11/3, Matrix Concatenate6/3  "0"
  2/1 -> Matrix Concatenate6/1, Matrix Concatenate9/2  "1"
  Demux/2 -> Matrix Concatenate11/2, Matrix Concatenate10/1  "a2"
  Demux/4 -> Matrix Concatenate10/3, Matrix Concatenate11/4  "b2"
  Demux/1 -> Matrix Concatenate9/1, Matrix Concatenate10/2  "a1"
  Matrix Concatenate14/1 -> M1/1
  Demux/3 -> Matrix Concatenate9/3, Matrix Concatenate10/4  "b1"
  In1/1 -> Demux/1

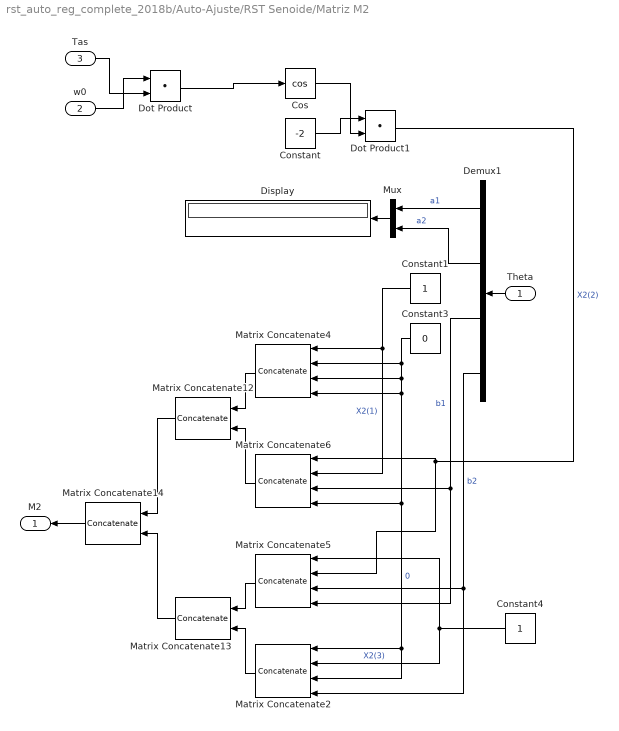
== system rst_auto_reg_complete_2018b/Auto-Ajuste/RST Senoide/Matriz M2 ==
  Theta : Inport
  w0 : Inport  Port=2
  Tas : Inport  Port=3
  Constant : Constant  Value=-2
  Constant1 : Constant
  Constant3 : Constant  Value=0
  Constant4 : Constant
  Cos : Trigonometry  Operator=cos
  Demux1 : Demux
  Display : Display
  Dot Product : DotProduct  InputSameDT=on  OutDataTypeStr=Inherit: Inherit via internal rule
  Dot Product1 : DotProduct  InputSameDT=on  OutDataTypeStr=Inherit: Inherit via internal rule
  Matrix Concatenate12 : Concatenate  Mode=Multidimensional array
  Matrix Concatenate13 : Concatenate  Mode=Multidimensional array
  Matrix Concatenate14 : Concatenate  Mode=Multidimensional array
  Matrix Concatenate{2,4..6} (4 alike) : Concatenate  NumInputs=4  Mode=Multidimensional array  ConcatenateDimension=2
  Mux : Mux  Inputs=2
  M2 : Outport
  wires:
  Constant/1 -> Dot Product1/1
  Cos/1 -> Dot Product1/2
  Matrix Concatenate6/1 -> Matrix Concatenate12/2
  Demux1/2 -> Mux/2  "a2"
  Dot Product/1 -> Cos/1
  Tas/1 -> Dot Product/2
  w0/1 -> Dot Product/1
  Theta/1 -> Demux1/1
  Demux1/1 -> Mux/1  "a1"
  Constant1/1 -> Matrix Concatenate6/2, Matrix Concatenate4/1  "X2(1)"
  Constant3/1 -> Matrix Concatenate4/3, Matrix Concatenate2/3, Matrix Concatenate2/1, Matrix Concatenate6/4, Matrix Concatenate4/4, Matrix Concatenate4/2  "0"
  Dot Product1/1 -> Matrix Concatenate5/2, Matrix Concatenate6/1  "X2(2)"
  Constant4/1 -> Matrix Concatenate5/1, Matrix Concatenate2/2  "X2(3)"
  Demux1/3 -> Matrix Concatenate5/4, Matrix Concatenate6/3  "b1"
  Demux1/4 -> Matrix Concatenate2/4, Matrix Concatenate5/3  "b2"
  Matrix Concatenate14/1 -> M2/1
  Matrix Concatenate13/1 -> Matrix Concatenate14/2
  Matrix Concatenate12/1 -> Matrix Concatenate14/1
  Matrix Concatenate4/1 -> Matrix Concatenate12/1
  Matrix Concatenate5/1 -> Matrix Concatenate13/1
  Matrix Concatenate2/1 -> Matrix Concatenate13/2
  Mux/1 -> Display/1

== system rst_auto_reg_complete_2018b/Auto-Ajuste/RST Senoide/Matriz Q1 ==
  P1 : Inport
  P2 : Inport  Port=2
  Constant : Constant
  Constant1 : Constant  Value=0
  Matrix Concatenate1 : Concatenate  Mode=Multidimensional array
  Matrix Concatenate2 : Concatenate  Mode=Multidimensional array
  Matrix Concatenate3 : Concatenate  Mode=Multidimensional array
  Q1 : Outport
  wires:
  Constant1/1 -> Matrix Concatenate3/2
  Constant/1 -> Matrix Concatenate1/1
  P1/1 -> Matrix Concatenate1/2
  P2/1 -> Matrix Concatenate3/1
  Matrix Concatenate3/1 -> Matrix Concatenate2/2
  Matrix Concatenate2/1 -> Q1/1
  Matrix Concatenate1/1 -> Matrix Concatenate2/1
